simulink model "threeStateSM_signalBuilder"  (R2024b)
settings: Solver=VariableStepAuto  StartTime=0.0  StopTime=10.0  RelTol=1e-3
libraries: SignalEditorBlockLib x1
settings Model: Creator=optimus  LastModifiedBy=optimus

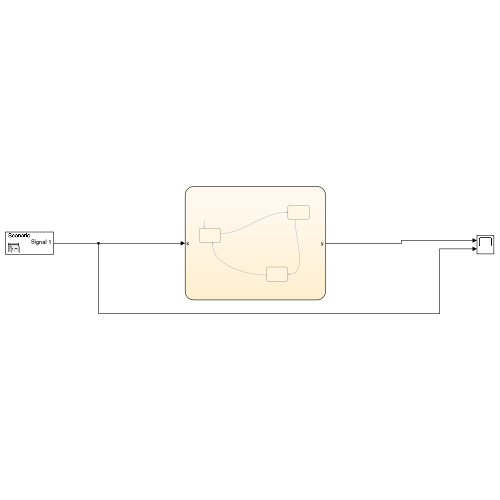
[thumbnail: Simulink's stored preview of the top-level diagram]
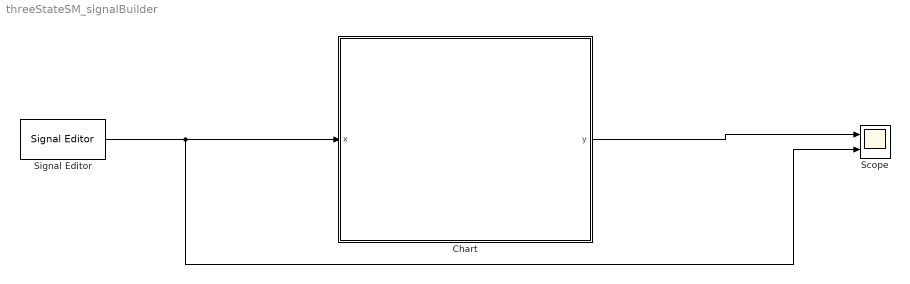
== system threeStateSM_signalBuilder ==
  Chart : Stateflow chart  TreatAsAtomicUnit=on
  Scope : Scope  NumInputPorts=2
  Signal Editor : SignalEditorBlockLib/Signal Editor  FileName=/Users/optimus/Documents/Matlab_Simulink_Projects/stateflow/signal_threeStateSM.mat  ActiveScenario=Scenario  ActiveSignal=Signal 1  IsBus=off  OutputBusObjectStr=Bus: BusObject  SampleTime=0  Interpolate=off  ZeroCross=off  OutputAfterFinalValue=Setting to zero  Unit=inherit  PreserveSignalName=on  ApplySigPropsToAllScenarios=on  ApplySigPropsToAllSignals=off
  wires:
  Signal Editor/1 -> Scope/2, Chart/1(x)
  Chart/1(y) -> Scope/1

== stateflow chart threeStateSM_signalBuilder/Chart ==
  state B
    entry:y=2;
  state A
    entry: y=1;
  state C
    entry:y=3;
  A -> B : [x>5]
  B -> C : [x==1]
  (default) -> A
  C -> A : [x<0]
  data: x input size=1; y output size=1
